simulink model "SENSORES"  (R2023b)
settings: Solver=VariableStepAuto  StartTime=0.0  StopTime=inf  RelTol=1e-3
libraries: arduinolib x5
settings Model: Creator=juanf  LastModifiedBy=juanf

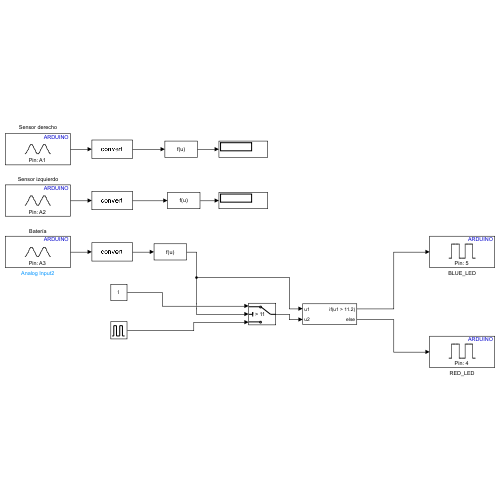
[thumbnail: Simulink's stored preview of the top-level diagram]
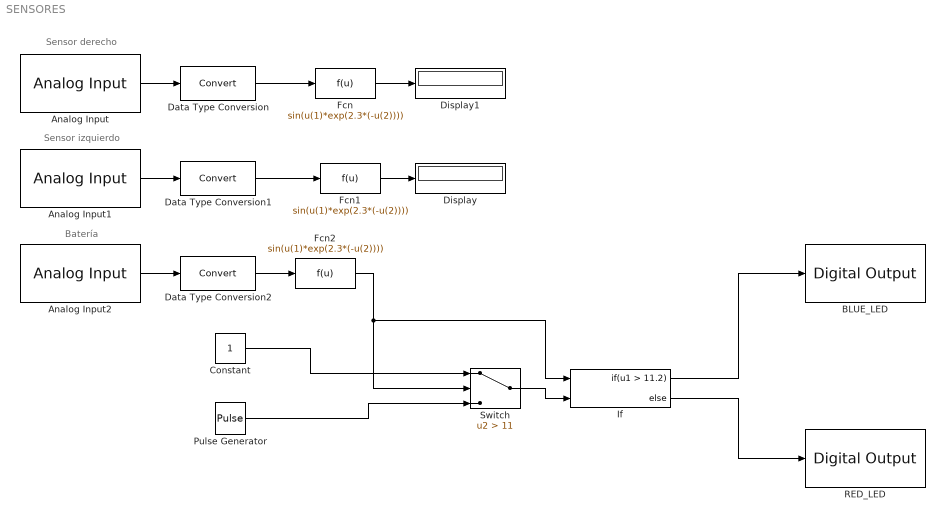
== system SENSORES ==
  note: Batería
  note: Sensor izquierdo
  note: Sensor derecho
  Analog Input : arduinolib/Analog Input  pinNumber=1  ReadResultsOnly=off  ConversionTriggerSource=Software  ExternalTriggerType=uint32( 0 )  OutputDataType=uint16  EnableConversionCompleteNotify=off  EnableOuputStatus=off  SampleTime=-1  blockPlatform=arduino
  Analog Input1 : arduinolib/Analog Input  pinNumber=2  ReadResultsOnly=off  ConversionTriggerSource=Software  ExternalTriggerType=uint32( 0 )  OutputDataType=uint16  EnableConversionCompleteNotify=off  EnableOuputStatus=off  SampleTime=-1  blockPlatform=arduino
  Analog Input2 : arduinolib/Analog Input  pinNumber=3  ReadResultsOnly=off  ConversionTriggerSource=Software  ExternalTriggerType=uint32( 0 )  OutputDataType=uint16  EnableConversionCompleteNotify=off  EnableOuputStatus=off  SampleTime=-1  blockPlatform=arduino
  BLUE_LED : arduinolib/Digital Output  pinNumber=5  Direction=output  blockPlatform=arduino
  Constant : Constant
  Data Type Conversion : DataTypeConversion  SaturateOnIntegerOverflow=off  RndMeth=Floor
  Data Type Conversion1 : DataTypeConversion  SaturateOnIntegerOverflow=off  RndMeth=Floor
  Data Type Conversion2 : DataTypeConversion  SaturateOnIntegerOverflow=off  RndMeth=Floor
  Display : Display
  Display1 : Display
  Fcn : Fcn  Expr=sin(u(1)*exp(2.3*(-u(2))))
  Fcn1 : Fcn  Expr=sin(u(1)*exp(2.3*(-u(2))))
  Fcn2 : Fcn  Expr=sin(u(1)*exp(2.3*(-u(2))))
  If : If  NumInputs=2  IfExpression=u1 > 11.2
  Pulse Generator : DiscretePulseGenerator  PulseType=Time based  Amplitude=15  Period=10  PulseWidth=5
  RED_LED : arduinolib/Digital Output  pinNumber=4  Direction=output  blockPlatform=arduino
  Switch : Switch  Criteria=u2 > Threshold  Threshold=11  SaturateOnIntegerOverflow=off  InputSameDT=off
  wires:
  Analog Input1/1 -> Data Type Conversion1/1
  Analog Input/1 -> Data Type Conversion/1
  Data Type Conversion/1 -> Fcn/1
  Data Type Conversion1/1 -> Fcn1/1
  Fcn/1 -> Display1/1
  Fcn1/1 -> Display/1
  Analog Input2/1 -> Data Type Conversion2/1
  Data Type Conversion2/1 -> Fcn2/1
  Fcn2/1 -> Switch/2, If/1
  Constant/1 -> Switch/1
  Pulse Generator/1 -> Switch/3
  Switch/1 -> If/2
  If/1 -> BLUE_LED/1
  If/2 -> RED_LED/1
